simulink model "OMSv1_5_lfd"  (Simulink 7.0)
settings: Solver=ode4  SolverMode=SingleTasking  StartTime=0.0  StopTime=4  FixedStep=0.001  MaxStep=0.001  RelTol=1e-3  AbsTol=1e-3
undefined symbols (not defined in the file): alexlaw, bs_onoff, bs_scale, bsfsacrit, bsfsvcrit, cnsgain, fs_onoff, fs_scale, fsdelaycalc, ltdrk, mdlparamlist, phasicgain, pmcgain, pmctau2, pmctau3, saccsw, spgain, tonicgain, tvrD, tvrN
(part 3 of 10)

== system OMSv1_5_lfd/OMS v1.4  12/31/07/PG w rNI2/PW funct ==
  note: This process continues until the error has been driven to zero or the input drops to zero,
      | and the integrator is reset and the pulse is ended.
  note: The input, scaled by the piece-wise linear function, is compared to the output of the
      | resettable integrator, which integrates a constant value each iteration.
  note: This block uses a resettable integrator and a piecewise-linear function (PWfunc) to generate
      | a pulse of appropriate duration for the incoming stimulus.
  note: (Init input:0)
  note: PW Function
  note: Last Modified
      | 08/17/07
  note: In order to produce exactly the same saccades in v1.4 as in 1.2 and 1.3, both using the old rNI,
      | we had to use a gain of 1.06 in the rNI path to set the smaller saccades equal
      | and change segments in the timing non-linearity (5-10)*1 and  (10-25)*2.05 and add (25-50)*2.1
  mcspl : Inport  OutDataType=sfix(16)  OutScaling=2^0
  Abs : Abs  SaturateOnIntegerOverflow=on
  Constant1 : Constant  Orientation=up  Value=0  OutDataType=sfix(16)  OutScaling=2^0
  Constant3 : Constant  Orientation=down  Value=1000  OutDataType=sfix(16)  OutScaling=2^0
  Gain : Gain  Orientation=left  Gain=1.06  ParameterDataType=sfix(16)  ParameterScaling=2^0  OutDataType=sfix(16)  OutScaling=2^0
  Good Reset Integrator1 : Subsystem  Orientation=left
      mask Display: disp('Resettable\nNI')
  Input Switch : Subsystem
      mask Display: disp('Input\nSwitch')
  Logical Operator : Logic  Orientation=left  Operator=OR
  Logical Operator1 : Logic  Orientation=up  Operator=NOT  Inputs=1
  PWfn : Lookup  Orientation=down  InputValues=[ 0, 0.1:5, 5:10, 10:25, 25:50 ]  Table="[ 0, (0.1:5)*0+15,  (5:10)*1+10,  (10:25)*2.05,  (25:50)*2.1]"  OutDataType=sfix(16)  OutScaling=2^0  SaturateOnIntegerOverflow=on
  Relational Operator1 : RelationalOperator  InputSameDT=on
  Relational Operator2 : RelationalOperator  Operator=<=  InputSameDT=on
  Sign : Subsystem
      mask Type: Sign
      mask Description: y = sign(x)
      mask Help: Sign Function:\n\t\t\ty = 1 if x > 0\n\t\t\ty = 0 if x = 0\n\t\t\ty = -1 if x < 0
      mask Display: plot(-50,-50,50,50,[-50,50],[0,0],[0,0],[-50,50],[-40,0],[-30,-30],[0,40],[30,30])
  Sum : Sum  Inputs=-+  OutDataType=sfix(16)  OutScaling=2^0  SaturateOnIntegerOverflow=on  InputSameDT=on
  dead zone : Constant  Orientation=up  Value=.04  OutDataType=sfix(16)  OutScaling=2^0
  loop breaker : Memory  Orientation=left
  out thresh : Constant  Value=0.2  OutDataType=sfix(16)  OutScaling=2^0
  pgw : Outport  OutDataType=sfix(16)  OutScaling=2^0  InitialOutput=0
  wires:
  Logical Operator1/1 -> Logical Operator/2
  Relational Operator1/1 -> Logical Operator1/1, Sign/1(in_1)
  Constant3/1 -> Good Reset Integrator1/1(input)
  Constant1/1 -> Good Reset Integrator1/3(initial condition)
  out thresh/1 -> Relational Operator1/2
  Input Switch/1(mcsw) -> Abs/1
  mcspl/1 -> Input Switch/1(mcspl)
  Sign/1(out_1) -> pgw/1, loop breaker/1
  Abs/1 -> PWfn/1, Relational Operator2/1
  PWfn/1 -> Sum/2
  Sum/1 -> Relational Operator1/1
  Logical Operator/1 -> Good Reset Integrator1/2(reset?)
  Good Reset Integrator1/1(out_1) -> Gain/1
  dead zone/1 -> Relational Operator2/2
  Relational Operator2/1 -> Logical Operator/1
  loop breaker/1 -> Input Switch/2(pgw)
  Gain/1 -> Sum/1

== system OMSv1_5_lfd/OMS v1.4  12/31/07/PG w rNI2/RefLatch (Default = 50ms) ==
  note: It's a cheap trick, but it seems to work:
  note: The falling edge" block's output becomes DISABLED upon
      | detection of the END of the input pulse, and remains
      | so until the refractory period of rp milliseconds has elapsed.
  note: By ANDing these outputs, we get a signal that is DISABLED
      | starting with the beginning of the input pulse, and remains so until
      | rp milliseconds after the termination of the pulse.
  note: The "NOT" gate outputs a DISABLE signal whenever there is any
      | input, so that there can be no response.
  in_1 : Inport  OutDataType=sfix(16)  OutScaling=2^0
  Abs : Abs  SaturateOnIntegerOverflow=on
  Logical Operator : Logic
  Logical Operator1 : Logic  Operator=NOT  Inputs=1
  trailing edge : Subsystem
      mask Display: disp('Refract\nLatch (te)')
  out_1 : Outport  OutDataType=sfix(16)  OutScaling=2^0  InitialOutput=0
  wires:
  Logical Operator/1 -> out_1/1
  Logical Operator1/1 -> Logical Operator/1
  trailing edge/1(out_1) -> Logical Operator/2
  Abs/1 -> Logical Operator1/1, trailing edge/1(in_1)
  in_1/1 -> Abs/1

== system OMSv1_5_lfd/OMS v1.4  12/31/07/PG w rNI2/SampHold?1 ==
  note: When "S/H?" is HIGH, then "Input" is switched directly to the
      | output ("sample").  When "S/H?" is LOW, the current output is
      | maintained ("hold").
  Input : Inport  OutDataType=sfix(16)  OutScaling=2^0
  S/H? : Inport  Port=2  OutDataType=sfix(16)  OutScaling=2^0
  Memory : Memory  Orientation=left
  Sign : Subsystem
      mask Type: Sign
      mask Description: y = sign(x)
      mask Help: Sign Function:\n\t\t\ty = 1 if x > 0\n\t\t\ty = 0 if x = 0\n\t\t\ty = -1 if x < 0
      mask Display: plot(-50,-50,50,50,[-50,50],[0,0],[0,0],[-50,50],[-40,0],[-30,-30],[0,40],[30,30])
  Switch2 : Switch  Threshold=0.5  SaturateOnIntegerOverflow=on  InputSameDT=on
  output : Outport  OutDataType=sfix(16)  OutScaling=2^0  InitialOutput=0
  wires:
  S/H?/1 -> Sign/1(in_1)
  Sign/1(out_1) -> Switch2/2
  Input/1 -> Switch2/1
  Switch2/1 -> output/1, Memory/1
  Memory/1 -> Switch2/3

== system OMSv1_5_lfd/OMS v1.4  12/31/07/oscillating PMC/NI Real3 ==
  note: Velocity Deadzone
  note: 12/10/07
  note: This block gets rid of the artifact at the beginning of the simulation
      | (the ripples) for normal simulation.
      | When there is a target velocity, or under Nystagmus condition, no deadzone should be applied.
  tvel : Inport  OutDataType=sfix(16)  OutScaling=2^0
  ecpyvel : Inport  Port=2  OutDataType=sfix(16)  OutScaling=2^0
  Boolify : Subsystem
      mask Display: disp('Boolify')
  Constant5 : Constant  Orientation=up  Value=2  OutDataType=sfix(16)  OutScaling=2^0
  Logical Operator1 : Logic  Operator=OR
  NI hold : Switch  Threshold=0.05  SaturateOnIntegerOverflow=on  InputSameDT=on
  Relational Operator : RelationalOperator  InputSameDT=on
  oppose2 : Constant  Orientation=up  Value=0  OutDataType=sfix(16)  OutScaling=2^0
  oppose7 : Constant  Value=mdlparamlist(1)  OutDataType=sfix(16)  OutScaling=2^0
  ecpyveldz : Outport  OutDataType=sfix(16)  OutScaling=2^0  InitialOutput=0
  wires:
  tvel/1 -> Boolify/1(In1)
  Boolify/1(Out1) -> Logical Operator1/1
  Constant5/1 -> Relational Operator/2
  oppose7/1 -> Relational Operator/1
  Relational Operator/1 -> Logical Operator1/2
  Logical Operator1/1 -> NI hold/2
  oppose2/1 -> NI hold/3
  ecpyvel/1 -> NI hold/1
  NI hold/1 -> ecpyveldz/1

== system OMSv1_5_lfd/OMS v1.4  12/31/07/Fixation/35 /Latch1 ==
  in_1 : Inport  OutDataType=sfix(16)  OutScaling=2^0
  in_2 : Inport  Port=2  OutDataType=sfix(16)  OutScaling=2^0
  Demux : Demux  Outputs=2
  Logic : CombinatorialLogic  TruthTable=[0 1;0 1;1 0;0 1;1 0;0 1;1 0;1 0]
  Memory : Memory  Orientation=left  X0=ini
  Mux : Mux  Inputs=3
  out_1 : Outport  OutDataType=sfix(16)  OutScaling=2^0  InitialOutput=0
  out_2 : Outport  Port=2  OutDataType=sfix(16)  OutScaling=2^0  InitialOutput=0
  wires:
  in_2/1 -> Mux/3
  in_1/1 -> Mux/2
  Memory/1 -> Mux/1
  Demux/1 -> Memory/1, out_1/1
  Mux/1 -> Logic/1
  Logic/1 -> Demux/1
  Demux/2 -> out_2/1

== system OMSv1_5_lfd/OMS v1.4  12/31/07/Fixation/35 /SampHold?2 ==
  note: When "S/H?" is LOW, then "Input" is switched directly to the
      | output ("sample").  When "S/H?" is HIGH, the current output is
      | maintained ("hold").
  Input : Inport  OutDataType=sfix(16)  OutScaling=2^0
  S/H? : Inport  Port=2  OutDataType=sfix(16)  OutScaling=2^0
  Memory : Memory  Orientation=left
  Sign : Subsystem
      mask Type: Sign
      mask Description: y = sign(x)
      mask Help: Sign Function:\n\t\t\ty = 1 if x > 0\n\t\t\ty = 0 if x = 0\n\t\t\ty = -1 if x < 0
      mask Display: plot(-50,-50,50,50,[-50,50],[0,0],[0,0],[-50,50],[-40,0],[-30,-30],[0,40],[30,30])
  Switch2 : Switch  Threshold=0.5  SaturateOnIntegerOverflow=on  InputSameDT=on
  output : Outport  OutDataType=sfix(16)  OutScaling=2^0  InitialOutput=0
  wires:
  S/H?/1 -> Sign/1(in_1)
  Sign/1(out_1) -> Switch2/2
  Input/1 -> Switch2/3
  Switch2/1 -> Memory/1, output/1
  Memory/1 -> Switch2/1

== system OMSv1_5_lfd/OMS v1.4  12/31/07/Fixation/35 /leading edge detect ==
  note: leading edge detection
  in_1 : Inport  OutDataType=sfix(16)  OutScaling=2^0
  Abs : Abs  SaturateOnIntegerOverflow=on
  Derivative : Derivative
  Relational Operator : RelationalOperator  Operator===  InputSameDT=on
  Sign : Subsystem
      mask Type: Sign
      mask Description: y = sign(x)
      mask Help: Sign Function:\n\t\t\ty = 1 if x > 0\n\t\t\ty = 0 if x = 0\n\t\t\ty = -1 if x < 0
      mask Display: plot(-50,-50,50,50,[-50,50],[0,0],[0,0],[-50,50],[-40,0],[-30,-30],[0,40],[30,30])
  Threshold 1 : Constant  OutDataType=sfix(16)  OutScaling=2^0
  out_1 : Outport  OutDataType=sfix(16)  OutScaling=2^0  InitialOutput=0
  wires:
  in_1/1 -> Abs/1
  Relational Operator/1 -> out_1/1
  Threshold 1/1 -> Relational Operator/2
  Sign/1(out_1) -> Relational Operator/1
  Derivative/1 -> Sign/1(in_1)
  Abs/1 -> Derivative/1

== system OMSv1_5_lfd/OMS v1.4  12/31/07/Fixation/35 /trailing edge detect ==
  note: It is also possible to remove the SIGNUM function
      | and the '==', and replace them with a simple
      | switch with a threshold of (say) 150 or so.
  note: trailing edge detection
  in_1 : Inport  OutDataType=sfix(16)  OutScaling=2^0
  Abs : Abs  SaturateOnIntegerOverflow=on
  Derivative : Derivative
  Relational Operator : RelationalOperator  Operator===  InputSameDT=on
  Sign : Subsystem
      mask Type: Sign
      mask Description: y = sign(x)
      mask Help: Sign Function:\n\t\t\ty = 1 if x > 0\n\t\t\ty = 0 if x = 0\n\t\t\ty = -1 if x < 0
      mask Display: plot(-50,-50,50,50,[-50,50],[0,0],[0,0],[-50,50],[-40,0],[-30,-30],[0,40],[30,30])
  Threshold 1 : Constant  Value=-1  OutDataType=sfix(16)  OutScaling=2^0
  out_1 : Outport  OutDataType=sfix(16)  OutScaling=2^0  InitialOutput=0
  wires:
  Abs/1 -> Derivative/1
  Derivative/1 -> Sign/1(in_1)
  Sign/1(out_1) -> Relational Operator/1
  Threshold 1/1 -> Relational Operator/2
  Relational Operator/1 -> out_1/1
  in_1/1 -> Abs/1

== system OMSv1_5_lfd/OMS v1.4  12/31/07/Fixation/Boolify2/direction1 ==
  in_1 : Inport  OutDataType=sfix(16)  OutScaling=2^0
  Constant : Constant  Value=0  OutDataType=sfix(16)  OutScaling=2^0
  Relational Operator : RelationalOperator  Operator=>  InputSameDT=on
  Relational Operator1 : RelationalOperator  Operator=<  InputSameDT=on
  Sum : Sum  Inputs=+-  OutDataType=sfix(16)  OutScaling=2^0  SaturateOnIntegerOverflow=on  InputSameDT=on
  out_1 : Outport  OutDataType=sfix(16)  OutScaling=2^0  InitialOutput=0
  wires:
  in_1/1 -> Relational Operator/1, Relational Operator1/1
  Constant/1 -> Relational Operator1/2, Relational Operator/2
  Relational Operator1/1 -> Sum/2
  Relational Operator/1 -> Sum/1
  Sum/1 -> out_1/1

== system OMSv1_5_lfd/OMS v1.4  12/31/07/IM CN-LMLN/Alexander's Law/Boolify ==
  TI : Inport  OutDataType=sfix(16)  OutScaling=2^0
  Abs2 : Abs  SaturateOnIntegerOverflow=on
  direction1 : Subsystem
      mask Type: Sign
      mask Description: y = sign(x)
      mask Help: Sign Function:\n\t\t\ty = 1 if x > 0\n\t\t\ty = 0 if x = 0\n\t\t\ty = -1 if x < 0
      mask Display: plot(-50,-50,50,50,[-50,50],[0,0],[0,0],[-50,50],[-40,0],[-30,-30],[0,40],[30,30])
  Switch Control : Outport  OutDataType=sfix(16)  OutScaling=2^0  InitialOutput=0
  wires:
  direction1/1(out_1) -> Switch Control/1
  TI/1 -> Abs2/1
  Abs2/1 -> direction1/1(in_1)

== system OMSv1_5_lfd/OMS v1.4  12/31/07/IM CN-LMLN/Alexander's Law/Boolify1 ==
  TI : Inport  OutDataType=sfix(16)  OutScaling=2^0
  Abs2 : Abs  SaturateOnIntegerOverflow=on
  direction1 : Subsystem
      mask Type: Sign
      mask Description: y = sign(x)
      mask Help: Sign Function:\n\t\t\ty = 1 if x > 0\n\t\t\ty = 0 if x = 0\n\t\t\ty = -1 if x < 0
      mask Display: plot(-50,-50,50,50,[-50,50],[0,0],[0,0],[-50,50],[-40,0],[-30,-30],[0,40],[30,30])
  Switch Control : Outport  OutDataType=sfix(16)  OutScaling=2^0  InitialOutput=0
  wires:
  Abs2/1 -> direction1/1(in_1)
  TI/1 -> Abs2/1
  direction1/1(out_1) -> Switch Control/1

== system OMSv1_5_lfd/OMS v1.4  12/31/07/IM CN-LMLN/Alexander's Law/direction ==
  in_1 : Inport  OutDataType=sfix(16)  OutScaling=2^0
  Constant : Constant  Value=0  OutDataType=sfix(16)  OutScaling=2^0
  Relational Operator : RelationalOperator  Operator=>  InputSameDT=on
  Relational Operator1 : RelationalOperator  Operator=<  InputSameDT=on
  Sum : Sum  Inputs=+-  OutDataType=sfix(16)  OutScaling=2^0  SaturateOnIntegerOverflow=on  InputSameDT=on
  out_1 : Outport  OutDataType=sfix(16)  OutScaling=2^0  InitialOutput=0
  wires:
  in_1/1 -> Relational Operator/1, Relational Operator1/1
  Constant/1 -> Relational Operator1/2, Relational Operator/2
  Relational Operator1/1 -> Sum/2
  Relational Operator/1 -> Sum/1
  Sum/1 -> out_1/1

== system OMSv1_5_lfd/OMS v1.4  12/31/07/IM CN-LMLN/BS/FS Logic/BS Enable1 ==
  note: BS Enable
  note: This block allows a BS for up to xx ms (set by "timer value")
      | after the acceleration criterion is met (i.e., drops below threshold)
  note: last mod:
      | 12/08/99
  note: (Default = 40deg/sec^2)
  bsprod : Inport  OutDataType=sfix(16)  OutScaling=2^0
  "[evelpr]" : Inport  Port=2  OutDataType=sfix(16)  OutScaling=2^0
  Abs1 : Abs  SaturateOnIntegerOverflow=on
  BS Timing : Subsystem
      mask Display: disp('BS\nEnable\nTiming')
  Derivative : Derivative
      mask Display: disp('s')
  Relational Operator3 : RelationalOperator  Operator=<=  InputSameDT=on
  Switch4 : Switch  Threshold=.5  SaturateOnIntegerOverflow=on  InputSameDT=on
  To Workspace14 : ToWorkspace  VariableName=bscmpr  SaveFormat=Array
      settings: MaxDataPoints=10000
      mask Type: imsw1in
  To Workspace15 : ToWorkspace  VariableName=bsenab  SaveFormat=Array
      settings: MaxDataPoints=10000
      mask Type: imsw1in
  To Workspace16 : ToWorkspace  VariableName=bsaccel1  SaveFormat=Array
      settings: MaxDataPoints=10000
      mask Type: imsw1in
  "accel. thresh " : Constant  Orientation=up  Value=bsfsacrit  OutDataType=sfix(16)  OutScaling=2^0
  off : Constant  Orientation=up  Value=0  OutDataType=sfix(16)  OutScaling=2^0
  timer value : Constant  Orientation=up  Value=0.01  OutDataType=sfix(16)  OutScaling=2^0
  "[bsmc]" : Outport  OutDataType=sfix(16)  OutScaling=2^0  InitialOutput=0
  wires:
  Relational Operator3/1 -> To Workspace14/1, BS Timing/1(From  <= [cmpr])
  Derivative/1 -> To Workspace16/1, Abs1/1
  Abs1/1 -> Relational Operator3/1
  BS Timing/1("[bsenab]") -> To Workspace15/1, Switch4/2
  "[evelpr]"/1 -> Derivative/1
  off/1 -> Switch4/3
  bsprod/1 -> Switch4/1
  Switch4/1 -> "[bsmc]"/1
  timer value/1 -> BS Timing/2(timer dur)
  "accel. thresh "/1 -> Relational Operator3/2

== system OMSv1_5_lfd/OMS v1.4  12/31/07/IM CN-LMLN/BS/FS Logic/FS Enable ==
  note: This block allows a FS for up to xx ms (set by "timer value")
      | after the acceleration criterion is met (i.e., drops below threshold)
  note: FS Enable
  note: last mod:
      | 07/03/07
  note: (Default = 40deg/sec^2)
  note: The prolonged fsbs? signal prevents fs during SP when they should be bs
  fsprod : Inport  OutDataType=sfix(16)  OutScaling=2^0
  "[evelpr]" : Inport  Port=2  OutDataType=sfix(16)  OutScaling=2^0
  fsbs? : Inport  Port=3  OutDataType=sfix(16)  OutScaling=2^0
  Abs1 : Abs  SaturateOnIntegerOverflow=on
  Derivative : Derivative
      mask Display: disp('s')
  FS Timing : Subsystem
      mask Display: disp('FS\nEnable\nTiming')
  Product8 : Product  OutDataType=sfix(16)  OutScaling=2^0  SaturateOnIntegerOverflow=on  RndMeth=Zero  InputSameDT=on
  Relational Operator3 : RelationalOperator  Operator=<=  InputSameDT=on
  SampHold?1 : Subsystem
      mask Display: disp('S=L\nH=H')
  Switch4 : Switch  Threshold=.5  SaturateOnIntegerOverflow=on  InputSameDT=on
  To Workspace16 : ToWorkspace  VariableName=fsaccel  SaveFormat=Array
      settings: MaxDataPoints=10000
      mask Type: imsw1in
  To Workspace17 : ToWorkspace  VariableName=fsenab  SaveFormat=Array
      settings: MaxDataPoints=10000
      mask Type: imsw1in
  accel. thresh : Constant  Orientation=up  Value=bsfsacrit  OutDataType=sfix(16)  OutScaling=2^0
  off : Constant  Orientation=up  Value=0  OutDataType=sfix(16)  OutScaling=2^0
  prolong : Subsystem  mask{prolong=5}
      mask prompts: prolong "Prolong pulse by?  (msec)"
      mask Display: disp('prolong')
  timer value : Constant  Orientation=up  Value=0.01  OutDataType=sfix(16)  OutScaling=2^0
  "[fsmc]" : Outport  OutDataType=sfix(16)  OutScaling=2^0  InitialOutput=0
  wires:
  timer value/1 -> FS Timing/2(timer dur)
  accel. thresh/1 -> Relational Operator3/2
  "[evelpr]"/1 -> Derivative/1
  FS Timing/1("[fsenab]") -> Product8/1
  Abs1/1 -> Relational Operator3/1
  Derivative/1 -> Abs1/1, To Workspace16/1
  fsprod/1 -> SampHold?1/1(Input)
  Switch4/1 -> "[fsmc]"/1
  off/1 -> Switch4/3
  SampHold?1/1(output) -> Switch4/1
  Relational Operator3/1 -> FS Timing/1(From  <= [cmpr])
  fsbs?/1 -> prolong/1(value(in))
  Product8/1 -> Switch4/2, SampHold?1/2(S/H?), To Workspace17/1
  prolong/1(value(out)) -> Product8/2

== system OMSv1_5_lfd/OMS v1.4  12/31/07/IM CN-LMLN/BS/FS Logic/FS or BS? ==
  note: The position error is compared to its value 3 milliseconds earlier.
      | If the error is _increasing_, we want to make a braking
      | saccade to oppose the runaway.
  note: If the position error is _decreasing_, then the eye is approaching the
      | target, and we would like to generate a foveating saccade, since
      | this is our best time to consider capturing the target.
  note: FS or BS?
  note: use diff & filter?
  pos error [ecd1str] : Inport  OutDataType=sfix(16)  OutScaling=2^0
  pgout : Inport  Port=2  OutDataType=sfix(16)  OutScaling=2^0
  Abs : Abs  SaturateOnIntegerOverflow=on
  Boolify : Subsystem
      mask Display: disp('Boolify')
  Relational Operator : RelationalOperator  Operator=>  InputSameDT=on
  SampHold?1 : Subsystem
      mask Display: disp('S&H\n(S=L)\n(H=H)')
  Transport Delay1 : TransportDelay  DelayTime=.002
      mask Display: disp('2ms')
  BS=1 FS=0 : Outport  OutDataType=sfix(16)  OutScaling=2^0  InitialOutput=0
  wires:
  Transport Delay1/1 -> Relational Operator/2
  pos error [ecd1str]/1 -> Abs/1
  Abs/1 -> Relational Operator/1, Transport Delay1/1
  pgout/1 -> Boolify/1(In1)
  Relational Operator/1 -> SampHold?1/1(Input)
  SampHold?1/1(output) -> BS=1 FS=0/1
  Boolify/1(Out1) -> SampHold?1/2(S/H?)

== system OMSv1_5_lfd/OMS v1.4  12/31/07/IM CN-LMLN/BS/FS Logic/TCHNG Override ==
  note: (FF init state: Q=1)
  note: * Leading Edge of input ENABLEs output
  note: Operation:
  note: *FS Enabling is initially DISABLED
  note: * Output of TIMER circuit DISABLES output
  note: TCHNG Override
  "[tchng]" : Inport  OutDataType=sfix(16)  OutScaling=2^0
  timer dur : Inport  Orientation=up  Port=2  OutDataType=sfix(16)  OutScaling=2^0
  Latch1 : Subsystem  mask(Latch){@1=1}
      mask prompts: @1 "Initial State for Output "Q":"
      mask help: Latch
      mask init:
      | ini=(@1~=0);
      mask Help: Latches the S input.  When S (set) is one, the Q output  becomes one.  The output remains one until the R (reset) input becomes one, forcing the output to zero.  If both R and S are one, the latch will be in an undefined state.
      mask Display: disp('S   Q\n\nR  !Q')
  Terminator : Terminator
  To Workspace13 : ToWorkspace  VariableName=tchngovr  SaveFormat=Array
      settings: Orientation=down  MaxDataPoints=10000
  event timer2 : Subsystem
      mask Display: disp('Event\nTimer2')
  leading edge detect : Subsystem
      mask Display: disp('Leading\nEdge Det')
  tchng sw : Outport  OutDataType=sfix(16)  OutScaling=2^0  InitialOutput=0
  wires:
  "[tchng]"/1 -> leading edge detect/1(in_1), event timer2/1(_PG)
  timer dur/1 -> event timer2/2(_timer value (port))
  event timer2/1(out_1) -> Latch1/1(in_1)
  leading edge detect/1(out_1) -> Latch1/2(in_2)
  Latch1/1(out_1) -> tchng sw/1, To Workspace13/1
  Latch1/2(out_2) -> Terminator/1

== system OMSv1_5_lfd/OMS v1.4  12/31/07/IM CN-LMLN/BS/FS Logic/direction ==
  in_1 : Inport  OutDataType=sfix(16)  OutScaling=2^0
  Constant : Constant  Value=0  OutDataType=sfix(16)  OutScaling=2^0
  Relational Operator : RelationalOperator  Operator=>  InputSameDT=on
  Relational Operator1 : RelationalOperator  Operator=<  InputSameDT=on
  Sum : Sum  Inputs=+-  OutDataType=sfix(16)  OutScaling=2^0  SaturateOnIntegerOverflow=on  InputSameDT=on
  out_1 : Outport  OutDataType=sfix(16)  OutScaling=2^0  InitialOutput=0
  wires:
  in_1/1 -> Relational Operator/1, Relational Operator1/1
  Constant/1 -> Relational Operator1/2, Relational Operator/2
  Relational Operator1/1 -> Sum/2
  Relational Operator/1 -> Sum/1
  Sum/1 -> out_1/1

== system OMSv1_5_lfd/OMS v1.4  12/31/07/IM CN-LMLN/BS/FS Logic/direction1 ==
  in_1 : Inport  OutDataType=sfix(16)  OutScaling=2^0
  Constant : Constant  Value=0  OutDataType=sfix(16)  OutScaling=2^0
  Relational Operator : RelationalOperator  Operator=>  InputSameDT=on
  Relational Operator1 : RelationalOperator  Operator=<  InputSameDT=on
  Sum : Sum  Inputs=+-  OutDataType=sfix(16)  OutScaling=2^0  SaturateOnIntegerOverflow=on  InputSameDT=on
  out_1 : Outport  OutDataType=sfix(16)  OutScaling=2^0  InitialOutput=0
  wires:
  in_1/1 -> Relational Operator/1, Relational Operator1/1
  Constant/1 -> Relational Operator1/2, Relational Operator/2
  Relational Operator1/1 -> Sum/2
  Relational Operator/1 -> Sum/1
  Sum/1 -> out_1/1

== system OMSv1_5_lfd/OMS v1.4  12/31/07/IM CN-LMLN/BS/FS Logic/prolong ==
  note: init = 0
  note: init = 0
  note: 11/22/99
  note: The start of the input pulse causes the value on input 1 to be held starting when the leading
      | edge occurs, and this value remains latched until 'delay' seconds after the pulse ends (trailing edge).
  note: The one integration step delay before the S&H block's S/H (bottom) input insures
      | that the input value to be latched is available to theS&H block's top input
      | before the S&H block tries to 'hold'.
  note: Stretch the duration of an input pulse, latching it at its value at pulse onset.
  note: init Q = 0
  value(in) : Inport  OutDataType=sfix(16)  OutScaling=2^0
  " x/1000" : Constant  Orientation=up  Value=0.001  OutDataType=sfix(16)  OutScaling=2^0
  Latch1 : Subsystem  mask(Latch){@1=0}
      mask prompts: @1 "Initial State for Output "Q":"
      mask help: Latch
      mask init:
      | ini=(@1~=0);
      mask Help: Latches the S input.  When S (set) is one, the Q output  becomes one.  The output remains one until the R (reset) input becomes one, forcing the output to zero.  If both R and S are one, the latch will be in an undefined state.
      mask Display: disp('S   Q\n\nR  !Q')
  Product : Product  OutDataType=sfix(16)  OutScaling=2^0  SaturateOnIntegerOverflow=on  RndMeth=Zero  InputSameDT=on
  SampHold?2 : Subsystem
      mask Display: disp('S=L\nH=H')
  Terminator : Terminator
      settings: Orientation=down
  Variable Transport Delay : VariableTransportDelay  MaximumDelay=10  MaximumPoints=prolong_buffersize
  leading edge detect : Subsystem
      mask Display: disp('Leading\nEdge Det')
  loop breaker2 : Memory
  stretch : Constant  Value=prolong  OutDataType=sfix(16)  OutScaling=2^0
  trailing edge detect : Subsystem
      mask Display: disp('Trailing\nEdge Det')
  value(out) : Outport  OutDataType=sfix(16)  OutScaling=2^0  InitialOutput=0
  wires:
  " x/1000"/1 -> Product/2
  Product/1 -> Variable Transport Delay/2
  stretch/1 -> Product/1
  loop breaker2/1 -> SampHold?2/2(S/H?)
  SampHold?2/1(output) -> value(out)/1
  Latch1/1(out_1) -> loop breaker2/1
  leading edge detect/1(out_1) -> Latch1/1(in_1)
  trailing edge detect/1(out_1) -> Variable Transport Delay/1
  Variable Transport Delay/1 -> Latch1/2(in_2)
  value(in)/1 -> SampHold?2/1(Input), trailing edge detect/1(in_1), leading edge detect/1(in_1)
  Latch1/2(out_2) -> Terminator/1

== system OMSv1_5_lfd/OMS v1.4  12/31/07/IM CN-LMLN/MdlPlnt+2/NI Real2 ==
  note: tenot
      |  reduction
      | coefficient
  note: Plant
  note: 06/14/2007
  fast components : Inport  OutDataType=sfix(16)  OutScaling=2^0
  slow components : Inport  Port=2  OutDataType=sfix(16)  OutScaling=2^0
  2-pole Plant1 : ZeroPole  Zeros=[ ]  Poles=[ -1/.18 -1/.007]  Gain=[1/.18 * 1/.007]
      mask Display: disp('2-pole\nPlant')
  Sum6 : Sum  OutDataType=sfix(16)  OutScaling=2^0  SaturateOnIntegerOverflow=on  InputSameDT=on
  xx4 : Gain  Gain=1-2*mdlparamlist(25)  ParameterDataType=sfix(16)  ParameterScaling=2^0  OutDataType=sfix(16)  OutScaling=2^0  SaturateOnIntegerOverflow=on
  ecpyy : Outport  OutDataType=sfix(16)  OutScaling=2^0
  wires:
  Sum6/1 -> 2-pole Plant1/1
  fast components/1 -> Sum6/1
  2-pole Plant1/1 -> ecpyy/1
  slow components/1 -> xx4/1
  xx4/1 -> Sum6/2

== system OMSv1_5_lfd/OMS v1.4  12/31/07/IM CN-LMLN/MdlPlnt+2/OMN1 ==
  note: Slow OMN
  note: 06/13/2007
  "[epossp]" : Inport  OutDataType=sfix(16)  OutScaling=2^0
  xx3 : Gain  ParameterDataType=sfix(16)  ParameterScaling=2^0  OutDataType=sfix(16)  OutScaling=2^0  SaturateOnIntegerOverflow=on
  "[psout]" : Outport  OutDataType=sfix(16)  OutScaling=2^0  InitialOutput=0
  wires:
  "[epossp]"/1 -> xx3/1
  xx3/1 -> "[psout]"/1

== system OMSv1_5_lfd/OMS v1.4  12/31/07/IM CN-LMLN/MdlPlnt+2/OMN3 ==
  note: Fast OMN
  note: Note that the OMN properly combines the pulse with the output of the NI, by latching
      | that output to its value at the moment the pulse appears.
  note: Operation: when the pulse is active ("from PG") it activates the switch, passing the
      | upper input through to the output.  When the pulse is over, the switch changes,
      | allowing the lower input (from the NI) to pass.
  note: This block behaves like the ocular motor neurons,combining a phasic pulse (from PG)
      | with the tonic step produced by integration of the step, yielding a Pulse-Step
      | to drive the plant.
  note: 06/13/2007
  "[epossp]" : Inport  OutDataType=sfix(16)  OutScaling=2^0
  "[pgout]" : Inport  Port=2  OutDataType=sfix(16)  OutScaling=2^0
  Abs : Abs  SaturateOnIntegerOverflow=on
  Gain _ : Gain  Gain=1.0  ParameterDataType=sfix(16)  ParameterScaling=2^0  OutDataType=sfix(16)  OutScaling=2^0  SaturateOnIntegerOverflow=on
  SampHold? : Subsystem
      mask Display: disp('H=H\nS=L')
  Sign : Subsystem
      mask Type: Sign
      mask Description: y = sign(x)
      mask Help: Sign Function:\n\t\t\ty = 1 if x > 0\n\t\t\ty = 0 if x = 0\n\t\t\ty = -1 if x < 0
      mask Display: plot(-50,-50,50,50,[-50,50],[0,0],[0,0],[-50,50],[-40,0],[-30,-30],[0,40],[30,30])
  Sum : Sum  OutDataType=sfix(16)  OutScaling=2^0  SaturateOnIntegerOverflow=on  InputSameDT=on
  Switch : Switch  Threshold=.5  SaturateOnIntegerOverflow=on  InputSameDT=on
  xx3 : Gain  ParameterDataType=sfix(16)  ParameterScaling=2^0  OutDataType=sfix(16)  OutScaling=2^0  SaturateOnIntegerOverflow=on
  "[psout]" : Outport  OutDataType=sfix(16)  OutScaling=2^0  InitialOutput=0
  wires:
  "[epossp]"/1 -> xx3/1
  Sign/1(out_1) -> Switch/2, SampHold?/2(S/H?)
  Gain _/1 -> Sum/1
  SampHold?/1(output) -> Sum/2
  Sum/1 -> Switch/1
  "[pgout]"/1 -> Gain _/1, Abs/1
  Switch/1 -> "[psout]"/1
  Abs/1 -> Sign/1(in_1)
  xx3/1 -> Switch/3, SampHold?/1(Input)

== system OMSv1_5_lfd/OMS v1.4  12/31/07/IM CN-LMLN/NI Control/Boolify ==
  In1 : Inport  OutDataType=sfix(16)  OutScaling=2^0
  Abs2 : Abs  SaturateOnIntegerOverflow=on
  direction1 : Subsystem
      mask Type: Sign
      mask Description: y = sign(x)
      mask Help: Sign Function:\n\t\t\ty = 1 if x > 0\n\t\t\ty = 0 if x = 0\n\t\t\ty = -1 if x < 0
      mask Display: plot(-50,-50,50,50,[-50,50],[0,0],[0,0],[-50,50],[-40,0],[-30,-30],[0,40],[30,30])
  Out1 : Outport  OutDataType=sfix(16)  OutScaling=2^0  InitialOutput=0
  wires:
  Abs2/1 -> direction1/1(in_1)
  In1/1 -> Abs2/1
  direction1/1(out_1) -> Out1/1

== system OMSv1_5_lfd/OMS v1.4  12/31/07/IM CN-LMLN/NI Control/Boolify1 ==
  In1 : Inport  OutDataType=sfix(16)  OutScaling=2^0
  Abs2 : Abs  SaturateOnIntegerOverflow=on
  direction1 : Subsystem
      mask Type: Sign
      mask Description: y = sign(x)
      mask Help: Sign Function:\n\t\t\ty = 1 if x > 0\n\t\t\ty = 0 if x = 0\n\t\t\ty = -1 if x < 0
      mask Display: plot(-50,-50,50,50,[-50,50],[0,0],[0,0],[-50,50],[-40,0],[-30,-30],[0,40],[30,30])
  Out1 : Outport  OutDataType=sfix(16)  OutScaling=2^0  InitialOutput=0
  wires:
  direction1/1(out_1) -> Out1/1
  In1/1 -> Abs2/1
  Abs2/1 -> direction1/1(in_1)

== system OMSv1_5_lfd/OMS v1.4  12/31/07/IM CN-LMLN/NI Control/Boolify2 ==
  In1 : Inport  OutDataType=sfix(16)  OutScaling=2^0
  Abs2 : Abs  SaturateOnIntegerOverflow=on
  direction1 : Subsystem
      mask Type: Sign
      mask Description: y = sign(x)
      mask Help: Sign Function:\n\t\t\ty = 1 if x > 0\n\t\t\ty = 0 if x = 0\n\t\t\ty = -1 if x < 0
      mask Display: plot(-50,-50,50,50,[-50,50],[0,0],[0,0],[-50,50],[-40,0],[-30,-30],[0,40],[30,30])
  Out1 : Outport  OutDataType=sfix(16)  OutScaling=2^0  InitialOutput=0
  wires:
  Abs2/1 -> direction1/1(in_1)
  In1/1 -> Abs2/1
  direction1/1(out_1) -> Out1/1

== system OMSv1_5_lfd/OMS v1.4  12/31/07/IM CN-LMLN/NI Control/Boolify3 ==
  In1 : Inport  OutDataType=sfix(16)  OutScaling=2^0
  Abs2 : Abs  SaturateOnIntegerOverflow=on
  direction1 : Subsystem
      mask Type: Sign
      mask Description: y = sign(x)
      mask Help: Sign Function:\n\t\t\ty = 1 if x > 0\n\t\t\ty = 0 if x = 0\n\t\t\ty = -1 if x < 0
      mask Display: plot(-50,-50,50,50,[-50,50],[0,0],[0,0],[-50,50],[-40,0],[-30,-30],[0,40],[30,30])
  Out1 : Outport  OutDataType=sfix(16)  OutScaling=2^0  InitialOutput=0
  wires:
  direction1/1(out_1) -> Out1/1
  In1/1 -> Abs2/1
  Abs2/1 -> direction1/1(in_1)

== system OMSv1_5_lfd/OMS v1.4  12/31/07/IM CN-LMLN/NI Control/DZ .5 ==
  note: We just output zero when the dead zone is in effect, and leave the
      |  output alone the rest of the time.
  note: This block is a better implementation of a dead zone than  the
      | block supplied by SIMULINK, because here we don't _subtract_
      | the dead zone from the rest of output.
  in_1 : Inport  OutDataType=sfix(16)  OutScaling=2^0
  Abs : Abs  Orientation=down  SaturateOnIntegerOverflow=on
  Relational Operator : RelationalOperator  InputSameDT=on
  Switch6 : Switch  Threshold=.5  SaturateOnIntegerOverflow=on  InputSameDT=on
  dead zone : Constant  Orientation=up  Value=.5  OutDataType=sfix(16)  OutScaling=2^0
  pos (deg) criterion1 : Constant  Orientation=left  Value=0  OutDataType=sfix(16)  OutScaling=2^0
  out_1 : Outport  OutDataType=sfix(16)  OutScaling=2^0  InitialOutput=0
  wires:
  Relational Operator/1 -> Switch6/2
  dead zone/1 -> Relational Operator/2
  pos (deg) criterion1/1 -> Switch6/3
  Abs/1 -> Relational Operator/1
  in_1/1 -> Switch6/1, Abs/1
  Switch6/1 -> out_1/1

== system OMSv1_5_lfd/OMS v1.4  12/31/07/IM CN-LMLN/NI Control/Latch1 ==
  in_1 : Inport  OutDataType=sfix(16)  OutScaling=2^0
  in_2 : Inport  Port=2  OutDataType=sfix(16)  OutScaling=2^0
  Demux : Demux  Outputs=2
  Logic : CombinatorialLogic  TruthTable=[0 1;0 1;1 0;0 1;1 0;0 1;1 0;1 0]
  Memory : Memory  Orientation=left  X0=ini
  Mux : Mux  Inputs=3
  out_1 : Outport  OutDataType=sfix(16)  OutScaling=2^0  InitialOutput=0
  out_2 : Outport  Port=2  OutDataType=sfix(16)  OutScaling=2^0  InitialOutput=0
  wires:
  in_2/1 -> Mux/3
  in_1/1 -> Mux/2
  Memory/1 -> Mux/1
  Demux/1 -> out_1/1, Memory/1
  Mux/1 -> Logic/1
  Logic/1 -> Demux/1
  Demux/2 -> out_2/1

== system OMSv1_5_lfd/OMS v1.4  12/31/07/IM CN-LMLN/NI Control/Latch2 ==
  in_1 : Inport  OutDataType=sfix(16)  OutScaling=2^0
  in_2 : Inport  Port=2  OutDataType=sfix(16)  OutScaling=2^0
  Demux : Demux  Outputs=2
  Logic : CombinatorialLogic  TruthTable=[0 1;0 1;1 0;0 1;1 0;0 1;1 0;1 0]
  Memory : Memory  Orientation=left  X0=ini
  Mux : Mux  Inputs=3
  out_1 : Outport  OutDataType=sfix(16)  OutScaling=2^0  InitialOutput=0
  out_2 : Outport  Port=2  OutDataType=sfix(16)  OutScaling=2^0  InitialOutput=0
  wires:
  Demux/2 -> out_2/1
  Logic/1 -> Demux/1
  Mux/1 -> Logic/1
  Demux/1 -> Memory/1, out_1/1
  Memory/1 -> Mux/1
  in_1/1 -> Mux/2
  in_2/1 -> Mux/3

== system OMSv1_5_lfd/OMS v1.4  12/31/07/IM CN-LMLN/NI Control/Zero-Cross ==
  note: Zero Cross Detect
  "[epr]" : Inport  OutDataType=sfix(16)  OutScaling=2^0
  Relational Operator : RelationalOperator  Operator=~=  InputSameDT=on
  Sign2 : Subsystem
      mask Type: Sign
      mask Description: y = sign(x)
      mask Help: Sign Function:\n\t\t\ty = 1 if x > 0\n\t\t\ty = 0 if x = 0\n\t\t\ty = -1 if x < 0
      mask Display: plot(-50,-50,50,50,[-50,50],[0,0],[0,0],[-50,50],[-40,0],[-30,-30],[0,40],[30,30])
  loop breaker1 : Memory
  "[epneq]" : Outport  OutDataType=sfix(16)  OutScaling=2^0  InitialOutput=0
  wires:
  Relational Operator/1 -> "[epneq]"/1
  loop breaker1/1 -> Relational Operator/2
  "[epr]"/1 -> Sign2/1(in_1)
  Sign2/1(out_1) -> Relational Operator/1, loop breaker1/1

== system OMSv1_5_lfd/OMS v1.4  12/31/07/IM CN-LMLN/NI Control/leading edge detect ==
  note: leading edge detection
  in_1 : Inport  OutDataType=sfix(16)  OutScaling=2^0
  Abs : Abs  SaturateOnIntegerOverflow=on
  Derivative : Derivative
  Relational Operator : RelationalOperator  Operator===  InputSameDT=on
  Sign : Subsystem
      mask Type: Sign
      mask Description: y = sign(x)
      mask Help: Sign Function:\n\t\t\ty = 1 if x > 0\n\t\t\ty = 0 if x = 0\n\t\t\ty = -1 if x < 0
      mask Display: plot(-50,-50,50,50,[-50,50],[0,0],[0,0],[-50,50],[-40,0],[-30,-30],[0,40],[30,30])
  Threshold 1 : Constant  OutDataType=sfix(16)  OutScaling=2^0
  out_1 : Outport  OutDataType=sfix(16)  OutScaling=2^0  InitialOutput=0
  wires:
  in_1/1 -> Abs/1
  Relational Operator/1 -> out_1/1
  Threshold 1/1 -> Relational Operator/2
  Sign/1(out_1) -> Relational Operator/1
  Derivative/1 -> Sign/1(in_1)
  Abs/1 -> Derivative/1

== system OMSv1_5_lfd/OMS v1.4  12/31/07/IM CN-LMLN/NI Control/leading edge detect1 ==
  note: leading edge detection
  in_1 : Inport  OutDataType=sfix(16)  OutScaling=2^0
  Abs : Abs  SaturateOnIntegerOverflow=on
  Derivative : Derivative
  Relational Operator : RelationalOperator  Operator===  InputSameDT=on
  Sign : Subsystem
      mask Type: Sign
      mask Description: y = sign(x)
      mask Help: Sign Function:\n\t\t\ty = 1 if x > 0\n\t\t\ty = 0 if x = 0\n\t\t\ty = -1 if x < 0
      mask Display: plot(-50,-50,50,50,[-50,50],[0,0],[0,0],[-50,50],[-40,0],[-30,-30],[0,40],[30,30])
  Threshold 1 : Constant  OutDataType=sfix(16)  OutScaling=2^0
  out_1 : Outport  OutDataType=sfix(16)  OutScaling=2^0  InitialOutput=0
  wires:
  Abs/1 -> Derivative/1
  Derivative/1 -> Sign/1(in_1)
  Sign/1(out_1) -> Relational Operator/1
  Threshold 1/1 -> Relational Operator/2
  Relational Operator/1 -> out_1/1
  in_1/1 -> Abs/1

== system OMSv1_5_lfd/OMS v1.4  12/31/07/IM CN-LMLN/NI Control/trailing edge detect ==
  note: It is also possible to remove the SIGNUM function
      | and the '==', and replace them with a simple
      | switch with a threshold of (say) 150 or so.
  note: trailing edge detection
  in_1 : Inport  OutDataType=sfix(16)  OutScaling=2^0
  Abs : Abs  SaturateOnIntegerOverflow=on
  Derivative : Derivative
  Relational Operator : RelationalOperator  Operator===  InputSameDT=on
  Sign : Subsystem
      mask Type: Sign
      mask Description: y = sign(x)
      mask Help: Sign Function:\n\t\t\ty = 1 if x > 0\n\t\t\ty = 0 if x = 0\n\t\t\ty = -1 if x < 0
      mask Display: plot(-50,-50,50,50,[-50,50],[0,0],[0,0],[-50,50],[-40,0],[-30,-30],[0,40],[30,30])
  Threshold 1 : Constant  Value=-1  OutDataType=sfix(16)  OutScaling=2^0
  out_1 : Outport  OutDataType=sfix(16)  OutScaling=2^0  InitialOutput=0
  wires:
  Abs/1 -> Derivative/1
  Derivative/1 -> Sign/1(in_1)
  Sign/1(out_1) -> Relational Operator/1
  Threshold 1/1 -> Relational Operator/2
  Relational Operator/1 -> out_1/1
  in_1/1 -> Abs/1

== system OMSv1_5_lfd/OMS v1.4  12/31/07/IM CN-LMLN/Sacc Blank/Latch1 ==
  in_1 : Inport  OutDataType=sfix(16)  OutScaling=2^0
  in_2 : Inport  Port=2  OutDataType=sfix(16)  OutScaling=2^0
  Demux : Demux  Outputs=2
  Logic : CombinatorialLogic  TruthTable=[0 1;0 1;1 0;0 1;1 0;0 1;1 0;1 0]
  Memory : Memory  Orientation=left  X0=ini
  Mux : Mux  Inputs=3
  out_1 : Outport  OutDataType=sfix(16)  OutScaling=2^0  InitialOutput=0
  out_2 : Outport  Port=2  OutDataType=sfix(16)  OutScaling=2^0  InitialOutput=0
  wires:
  Demux/2 -> out_2/1
  Logic/1 -> Demux/1
  Mux/1 -> Logic/1
  Demux/1 -> out_1/1, Memory/1
  Memory/1 -> Mux/1
  in_1/1 -> Mux/2
  in_2/1 -> Mux/3

== system OMSv1_5_lfd/OMS v1.4  12/31/07/IM CN-LMLN/Sacc Blank/Latch2 ==
  in_1 : Inport  OutDataType=sfix(16)  OutScaling=2^0
  in_2 : Inport  Port=2  OutDataType=sfix(16)  OutScaling=2^0
  Demux : Demux  Outputs=2
  Logic : CombinatorialLogic  TruthTable=[0 1;0 1;1 0;0 1;1 0;0 1;1 0;1 0]
  Memory : Memory  Orientation=left  X0=ini
  Mux : Mux  Inputs=3
  out_1 : Outport  OutDataType=sfix(16)  OutScaling=2^0  InitialOutput=0
  out_2 : Outport  Port=2  OutDataType=sfix(16)  OutScaling=2^0  InitialOutput=0
  wires:
  in_2/1 -> Mux/3
  in_1/1 -> Mux/2
  Memory/1 -> Mux/1
  Demux/1 -> Memory/1, out_1/1
  Mux/1 -> Logic/1
  Logic/1 -> Demux/1
  Demux/2 -> out_2/1

== system OMSv1_5_lfd/OMS v1.4  12/31/07/IM CN-LMLN/Sacc Blank/event timer1 ==
  note: In 2) Subsequent events DO NOT reset the counter; it only resets when it
      | reaches zero
  note: 2) A new event (leading or trailing edge) is detected. -- Only case 1)
  note: 1) The count reaches its limit (set in "timer value") -- Both case 1) and 2)
  note: In 1), Any event (leading or trailing edge) will reset the counter so that it
      | counts down from the end trailing edge) of that event.
  note: It has TWO modes: 1) Event resettable and 2) Event Non-resettable
  note: The real trick here is understanding how to reload the countdown.
      | It resets if either of two conditions is met:
  note: The "OR" gate allows either of these conditions to reset the circuit.  The delay before the
      | "S" input of the flip-flop prevents both "S" and "R" from being set simultaneously, because
      | this would put the flip-flop in an undefined state.
  note: Therefore, an event first RESETS and then SETS the flip-flop.
  note: (Init input: 0)
  note: (FF init state: Q=0)
  note: (Init input: 0)
  note: This block is an RESETTABLE EVENT TIMER.  It outputs a spike of unit height xx milliseconds
      | (set by "timer value") after it detects an event ( i.e a TRAILING edge which represents the end of a
      |  saccadic pulse)
  note: Resettable
      | Event Timer
  _PG : Inport  OutDataType=sfix(16)  OutScaling=2^0
  _timer value (port) : Inport  Port=2  OutDataType=sfix(16)  OutScaling=2^0
  1 msec : TransportDelay  DelayTime=.001
  Clock : Clock
      settings: Decimation=10
  Latch1 : Subsystem  mask(Latch){@1=0}
      mask prompts: @1 "Initial State for Output "Q":"
      mask help: Latch
      mask init:
      | ini=(@1~=0);
      mask Help: Latches the S input.  When S (set) is one, the Q output  becomes one.  The output remains one until the R (reset) input becomes one, forcing the output to zero.  If both R and S are one, the latch will be in an undefined state.
      mask Display: disp('S   Q\n\nR  !Q')
  Logical Operator : Logic  Operator=OR  Inputs=3
  Logical Operator1 : Logic
  Logical Operator2 : Logic
  Relational Operator : RelationalOperator  InputSameDT=on
  SampHold?1 : Subsystem
      mask Display: disp('S&H\n(S=L)\n(H=H)')
  Sum : Sum  Inputs=+-  OutDataType=sfix(16)  OutScaling=2^0  SaturateOnIntegerOverflow=on  InputSameDT=on
  Terminator : Terminator
  event resettable? : Constant  Orientation=up  OutDataType=sfix(16)  OutScaling=2^0
  leading edge detect : Subsystem
      mask Display: disp('Leading\nEdge Det')
  loop breaker : Memory  Orientation=left
  trailing edge detect : Subsystem
      mask Display: disp('Trailing\nEdge Det')
  out_1 : Outport  OutDataType=sfix(16)  OutScaling=2^0  InitialOutput=0
  wires:
  event resettable?/1 -> Logical Operator1/2, Logical Operator2/2
  leading edge detect/1(out_1) -> Logical Operator2/1
  Logical Operator2/1 -> Logical Operator/2
  trailing edge detect/1(out_1) -> 1 msec/1, Logical Operator1/1
  Logical Operator1/1 -> Logical Operator/1
  loop breaker/1 -> Logical Operator/3
  Latch1/1(out_1) -> SampHold?1/2(S/H?)
  Sum/1 -> Relational Operator/1
  Clock/1 -> SampHold?1/1(Input), Sum/1
  _PG/1 -> leading edge detect/1(in_1), trailing edge detect/1(in_1)
  Relational Operator/1 -> out_1/1, loop breaker/1
  SampHold?1/1(output) -> Sum/2
  Logical Operator/1 -> Latch1/2(in_2)
  1 msec/1 -> Latch1/1(in_1)
  _timer value (port)/1 -> Relational Operator/2
  Latch1/2(out_2) -> Terminator/1

== system OMSv1_5_lfd/OMS v1.4  12/31/07/IM CN-LMLN/Sacc Blank/leading edge detect ==
  note: leading edge detection
  in_1 : Inport  OutDataType=sfix(16)  OutScaling=2^0
  Abs : Abs  SaturateOnIntegerOverflow=on
  Derivative : Derivative
  Relational Operator : RelationalOperator  Operator===  InputSameDT=on
  Sign : Subsystem
      mask Type: Sign
      mask Description: y = sign(x)
      mask Help: Sign Function:\n\t\t\ty = 1 if x > 0\n\t\t\ty = 0 if x = 0\n\t\t\ty = -1 if x < 0
      mask Display: plot(-50,-50,50,50,[-50,50],[0,0],[0,0],[-50,50],[-40,0],[-30,-30],[0,40],[30,30])
  Threshold 1 : Constant  OutDataType=sfix(16)  OutScaling=2^0
  out_1 : Outport  OutDataType=sfix(16)  OutScaling=2^0  InitialOutput=0
  wires:
  Abs/1 -> Derivative/1
  Derivative/1 -> Sign/1(in_1)
  Sign/1(out_1) -> Relational Operator/1
  Threshold 1/1 -> Relational Operator/2
  Relational Operator/1 -> out_1/1
  in_1/1 -> Abs/1

== system OMSv1_5_lfd/OMS v1.4  12/31/07/IM CN-LMLN/Sacc Blank/rising edge detect ==
  note: rising edge detection
  in_1 : Inport  OutDataType=sfix(16)  OutScaling=2^0
  Derivative : Derivative
  Relational Operator : RelationalOperator  Operator===  InputSameDT=on
  Sign : Subsystem
      mask Type: Sign
      mask Description: y = sign(x)
      mask Help: Sign Function:\n\t\t\ty = 1 if x > 0\n\t\t\ty = 0 if x = 0\n\t\t\ty = -1 if x < 0
      mask Display: plot(-50,-50,50,50,[-50,50],[0,0],[0,0],[-50,50],[-40,0],[-30,-30],[0,40],[30,30])
  Threshold 1 : Constant  OutDataType=sfix(16)  OutScaling=2^0
  out_1 : Outport  OutDataType=sfix(16)  OutScaling=2^0  InitialOutput=0
  wires:
  Derivative/1 -> Sign/1(in_1)
  Sign/1(out_1) -> Relational Operator/1
  Threshold 1/1 -> Relational Operator/2
  Relational Operator/1 -> out_1/1
  in_1/1 -> Derivative/1

== system OMSv1_5_lfd/OMS v1.4  12/31/07/IM CN-LMLN/Sacc Blank/rising edge detect1 ==
  note: rising edge detection
  in_1 : Inport  OutDataType=sfix(16)  OutScaling=2^0
  Derivative : Derivative
  Relational Operator : RelationalOperator  Operator===  InputSameDT=on
  Sign : Subsystem
      mask Type: Sign
      mask Description: y = sign(x)
      mask Help: Sign Function:\n\t\t\ty = 1 if x > 0\n\t\t\ty = 0 if x = 0\n\t\t\ty = -1 if x < 0
      mask Display: plot(-50,-50,50,50,[-50,50],[0,0],[0,0],[-50,50],[-40,0],[-30,-30],[0,40],[30,30])
  Threshold 1 : Constant  OutDataType=sfix(16)  OutScaling=2^0
  out_1 : Outport  OutDataType=sfix(16)  OutScaling=2^0  InitialOutput=0
  wires:
  in_1/1 -> Derivative/1
  Relational Operator/1 -> out_1/1
  Threshold 1/1 -> Relational Operator/2
  Sign/1(out_1) -> Relational Operator/1
  Derivative/1 -> Sign/1(in_1)
